simulink subsystem "HMT_Controller"  (R2022b)
settings: Solver=VariableStepAuto  StartTime=0.0  StopTime=10.0  RelTol=1e-3
libraries: simulink x1
settings Model: Creator=david  LastModifiedBy=david

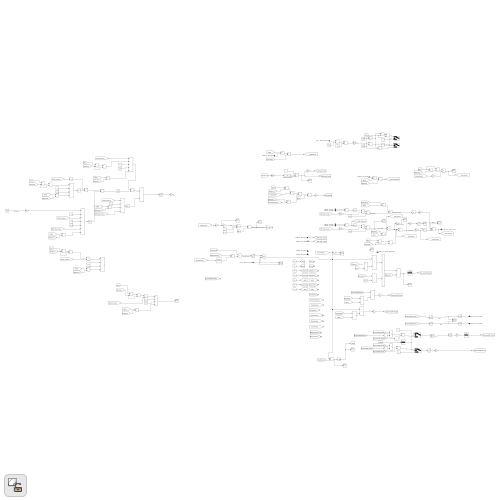
[thumbnail: Simulink's stored preview of the top-level diagram]
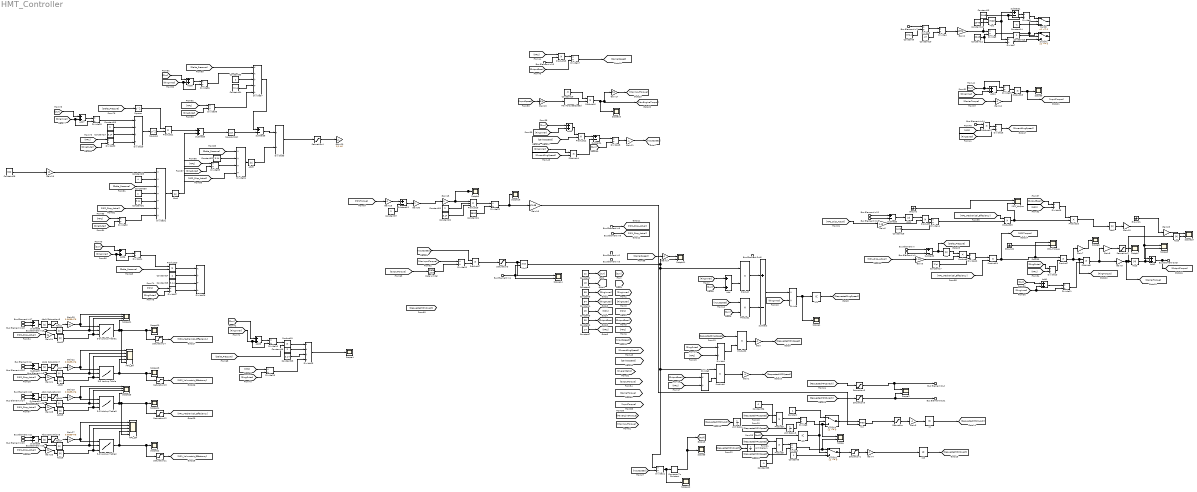
== system HMT_Controller ==
  Bus Element In{,6,12,17,21..22} (6 alike) : Inport  PortName=Feedback  Element=Pressure_A
  Bus Element In{1,10,13,18,23..24} (6 alike) : Inport  PortName=Feedback  Element=Pressure_B
  Bus Element In{2,14,25..26} (4 alike) : Inport  PortName=Feedback  Element=MP1_Speed
  Bus Element In{3,5,15,19} (4 alike) : Inport  PortName=Feedback  Element=MP2_Speed
  Bus Element In8 : Inport  PortName=Feedback  Element=MP1_Swash
  Bus Element In9 : Inport  PortName=Feedback  Element=MP2_Swash
  Bus Element In4 : Inport  Port=2  PortName=Control  Element=Speed_Command
  Bus Element In7 : Inport  Port=2  PortName=Control  Element=Speed_Command
  3-D Lookup Table : Lookup_n-D  NumberOfTableDimensions=3  BreakpointsForDimension1=[10,135,278]  BreakpointsForDimension2=[500,1974,4000]  BreakpointsForDimension3=[4.8,12,24]  Table=cat(3,[.47,0.01,0.01; .98,.38,.01;.98,.67,.38],[.81,.12,0.01;.99,.80,.65;1.00,.88,.79],[.93,.61,.42;1.00,.91,.85;1.00,.95,.89])  InterpMethod=Cubic spline  ExtrapMethod=Clip  UseLastTableValue=on  InternalRulePriority=Speed  RndMeth=Simplest
      settings: InputPortMap=u0,u1,u2
  3-D Lookup Table1 : Lookup_n-D  NumberOfTableDimensions=3  BreakpointsForDimension1=[10,135,278]  BreakpointsForDimension2=[500,1974,4000]  BreakpointsForDimension3=[4.8,12,24]  Table=cat(3,[.46,.62,.54;.27,.74,.83;.21,.73,.89],[.65,.86,.83;.46,.86,.94;.35,.86,.95],[.66,.83,.85;.53,.88,.91;.39,.87,.94])  InterpMethod=Cubic spline  ExtrapMethod=Clip  UseLastTableValue=on  InternalRulePriority=Speed  RndMeth=Simplest
      settings: InputPortMap=u0,u1,u2
  3-D Lookup Table2 : Lookup_n-D  NumberOfTableDimensions=3  BreakpointsForDimension1=[10,135,278]  BreakpointsForDimension2=[500,1974,4000]  BreakpointsForDimension3=[4.8,12,24]  Table=cat(3,[.47,0.01,0.01; .98,.38,.01;.98,.67,.38],[.81,.12,0.01;.99,.80,.65;1.00,.88,.79],[.93,.61,.42;1.00,.91,.85;1.00,.95,.89])  InterpMethod=Cubic spline  ExtrapMethod=Clip  UseLastTableValue=on  InternalRulePriority=Speed  RndMeth=Simplest
      settings: InputPortMap=u0,u1,u2
  3-D Lookup Table3 : Lookup_n-D  NumberOfTableDimensions=3  BreakpointsForDimension1=[10,135,278]  BreakpointsForDimension2=[500,1974,4000]  BreakpointsForDimension3=[4.8,12,24]  Table=cat(3,[.46,.62,.54;.27,.74,.83;.21,.73,.89],[.65,.86,.83;.46,.86,.94;.35,.86,.95],[.66,.83,.85;.53,.88,.91;.39,.87,.94])  InterpMethod=Cubic spline  ExtrapMethod=Clip  UseLastTableValue=on  InternalRulePriority=Speed  RndMeth=Simplest
      settings: InputPortMap=u0,u1,u2
  Abs{,1..18} (19 alike) : Abs  SaturateOnIntegerOverflow=off
  Add{,1..8} (9 alike) : Sum
  Compare To Constant : simulink/Logic and Bit Operations/Compare To Constant  relop=>=  const=.14389  OutDataTypeStr=boolean
  Constant : Constant
  Constant1 : Constant  Value=22
  Constant10 : Constant  Value=.27
  Constant11 : Constant  Value=2048
  Constant12 : Constant  Value=2048
  Constant13 : Constant  Value=2048
  Constant14 : Constant  Value=-1
  Constant15 : Constant
  Constant{16,20,24,26,30,33,37} (7 alike) : Constant  Value=2
  Constant17 : Constant  Value=2*pi
  Constant18 : Constant  Value=6.28
  Constant19 : Constant  Value=.8
  Constant2 : Constant  Value=18
  Constant21 : Constant  Value=3800
  Constant{22..23,25,27,31..32,34} (7 alike) : Constant  Value=3.14
  Constant28 : Constant  Value=300
  Constant29 : Constant  Value=4
  Constant3 : Constant  Value=58
  Constant35 : Constant  Value=-1
  Constant36 : Constant  Value=-1
  Constant4 : Constant  Value=54
  Constant5 : Constant  Value=25
  Constant6 : Constant  Value=38
  Constant7 : Constant  Value=14
  Constant8 : Constant
  Constant9 : Constant  Value=3724
  Divide{,1..22,24..25,27..28,30,32..33,35..36,38} (33 alike) : Product  Inputs=*/
  Divide{23,26,29,34} (4 alike) : Product  Inputs=*///
  Divide31 : Product  Inputs=***////
  Divide37 : Product  Inputs=**///
  Gain{,1,3..4,11..12,14,18} (8 alike) : Gain  Gain=-1
  Gain{8..10,23} (4 alike) : Gain  Gain=1/12
  Gain13 : Gain  Gain=3/4
  Gain15 : Gain
  Gain16 : Gain  Gain=1/1.46
  Gain17 : Gain  Gain=3/4
  Gain19 : Gain  Gain=12
  Gain2 : Gain  Gain=4096
  Gain20 : Gain  Gain=1/1.46
  Gain{21,24,26,28} (4 alike) : Gain  Gain=24
  Gain{22,25,27,29} (4 alike) : Gain  Gain=0.0689476
  Gain30 : Gain
  Gain5 : Gain  Gain=1.46
  Gain6 : Gain  Gain=1.46
  Gain7 : Gain  Gain=-1/12
  Ground : Ground
  Ground1 : Ground
  Ground2 : Ground
  IC : InitialCondition  Value=0
  IC1 : InitialCondition  Value=-1000
  IC2 : InitialCondition  Value=false
  IC3 : InitialCondition  Value=-1
  MP1_Eff : Scope  NumInputPorts=5
  MP1_Torque : Scope  NumInputPorts=2
  MP2_Eff : Scope  NumInputPorts=5
  MP2_torque : Scope  NumInputPorts=2
  MaxTorqueatSpeed : Fcn  Expr=-0.000019*u(1)^2 + 0.102035*u(1) - 80.132873
  Min : MinMax  Function=max  Inputs=2
  Min1 : MinMax  Inputs=2
  Mod : Math  Operator=mod
  Product{,1..17,19..21,23..24} (23 alike) : Product
  Product18 : Product  Inputs=3
  Rate Limiter : RateLimiter  RisingSlewLimit=inf  FallingSlewLimit=-inf  SampleTimeMode=inherited
  Saturation{,1,5..6} (4 alike) : Saturate  UpperLimit=1  LowerLimit=-1
  Saturation{7..10} (4 alike) : Saturate  UpperLimit=4000  LowerLimit=0
  Saturation{11..14} (4 alike) : Saturate  UpperLimit=1  LowerLimit=1
  Saturation2 : Saturate  UpperLimit=1000  LowerLimit=-1000
  Saturation3 : Saturate  UpperLimit=2000  LowerLimit=0
  Saturation4 : Saturate  UpperLimit=1.46  LowerLimit=-1.46
  Scope{,2,8,11,14,19} (6 alike) : Scope  NumInputPorts=2
  Scope{1,3..7,9..10,12..13,16,20,22,24} (14 alike) : Scope
  Scope21 : Scope  NumInputPorts=4
  Scope25 : Scope  NumInputPorts=4
  Square : Math  Operator=square
  Square Root : Sqrt
  Square1 : Math  Operator=square
  Subtract{,1..4,6..11} (11 alike) : Sum  Inputs=+-
  Subtract5 : Sum
  Switch : Switch  Criteria=u2 ~= 0  SaturateOnIntegerOverflow=off  InputSameDT=off
  Switch1 : Switch  Criteria=u2 ~= 0  SaturateOnIntegerOverflow=off  InputSameDT=off
  Switch2 : Switch  Criteria=u2 ~= 0  Threshold=688  SaturateOnIntegerOverflow=off  InputSameDT=off
  Switch3 : Switch  Criteria=u2 ~= 0  Threshold=688  SaturateOnIntegerOverflow=off  InputSameDT=off
  Unit Delay : UnitDelay  InitialCondition=1  SampleTime=-1  HasFrameUpgradeWarning=on
  Unit Delay1 : UnitDelay  SampleTime=-1  HasFrameUpgradeWarning=on
  Unit Delay3 : UnitDelay  InitialCondition=1  SampleTime=-1  HasFrameUpgradeWarning=on
  Bus Element Out : Outport  VectorParamsAs1DForOutWhenUnconnected=off  PortName=Control_Out  Element=MP1_Swash
  Bus Element Out1 : Outport  VectorParamsAs1DForOutWhenUnconnected=off  PortName=Control_Out  Element=MP2_Swash
  Bus Element Out2 : Outport  VectorParamsAs1DForOutWhenUnconnected=off  PortName=Control_Out  Element=Engine_Speed_CMD
  Bus Element Out3 : Outport  VectorParamsAs1DForOutWhenUnconnected=off  PortName=Control_Out  Element=Output_Torque
  wires:
  [OutputTorque] -> Rate Limiter/1
  Min1/1 -> Product/1, Product4/1, Divide21/1, Scope11/2
  Min/1 -> Saturation/1
  Saturation4/1 -> Gain20/1
  Abs5/1 -> Divide33/2
  Divide34/1 -> Abs5/1
  Abs4/1 -> Subtract5/2
  Divide37/1 -> Subtract6/1
  Subtract6/1 -> Divide33/1
  Square Root/1 -> Subtract6/2
  [MP1] -> Divide38/1
  [RingOuter] -> Divide38/2
  Divide38/1 -> Divide37/5
  Constant34/1 -> Divide37/4
  Constant33/1 -> Divide37/3
  [Delta_Pressure] -> Divide37/1
  Divide36/1 -> Divide37/2
  Add8/1 -> Divide36/1
  [RingInner] -> Divide36/2, Add8/2
  [Sun] -> Add8/1
  Gain19/1 -> Divide31/1
  Divide33/1 -> Saturation4/1
  [MP2_Disp_Actual] -> Divide34/4
  [MP1] -> Divide35/1
  [RingOuter] -> Divide35/2
  Divide35/1 -> Divide34/3
  Constant32/1 -> Divide34/2
  [Delta_Pressure] -> Divide34/1
  Subtract5/1 -> Square Root/1
  Divide31/1 -> Abs4/1
  Divide32/1 -> Divide31/7
  [RingOuter] -> Divide32/2
  [MP1] -> Divide32/1
  [MP2_Disp_Actual] -> Divide31/6
  Constant31/1 -> Divide31/5
  Constant30/1 -> Divide31/4
  Constant29/1 -> Divide31/2
  Constant28/1 -> Gain19/1  "Torque Limit"
  [Delta_Pressure] -> Divide31/3
  Product21/1 -> Subtract5/1
  Square/1 -> Product21/1
  Square1/1 -> Product21/2
  Divide29/1 -> Square1/1
  Divide28/1 -> Divide29/1
  [Sun] -> Add7/1
  [RingInner] -> Add7/2, Divide28/2
  Add7/1 -> Divide28/1
  Constant26/1 -> Divide29/2
  Constant27/1 -> Divide29/3
  Divide30/1 -> Divide29/4
  [RingOuter] -> Divide30/2
  [MP1] -> Divide30/1
  [Delta_Pressure] -> Square/1
  [MP1] -> Divide27/1
  [RingOuter] -> Divide27/2
  Divide27/1 -> Divide26/4
  Constant25/1 -> Divide26/3
  Constant24/1 -> Divide26/2
  Product20/1 -> Divide26/1
  [Delta_Pressure] -> Product20/2
  Divide24/1 -> Product20/1
  Add6/1 -> Divide24/1
  [RingInner] -> Divide24/2, Add6/2
  [Sun] -> Add6/1
  Constant1/1 -> [Sun]
  Constant2/1 -> [Planet]
  Constant4/1 -> [RingOuter]
  Constant3/1 -> [RingInner]
  Constant5/1 -> [MP1]
  Constant6/1 -> [OutputGear]
  Constant7/1 -> [MP2]
  [RingInner] -> Add/1
  [Sun] -> Add/2
  Add/1 -> Product/2
  [Sun] -> Product1/2
  Product1/1 -> Subtract/2
  Product/1 -> Subtract/1
  Subtract/1 -> Divide/1
  [RingInner] -> Divide/2
  [InputSpeed] -> Product1/1
  Divide/1 -> IC1/1, Scope1/1
  [RequestedRingSpeed] -> Product2/1
  [RingOuter] -> Divide1/1
  [MP1] -> Divide1/2
  Divide1/1 -> Product2/2
  Product2/1 -> Gain/1
  Gain/1 -> [RequestedMP1Speed]
  Divide2/1 -> Product4/2
  [OutputGear] -> Divide2/1
  [MP2] -> Divide2/2
  Gain1/1 -> [RequestedMP2Speed]
  Bus Element In7/1 -> Divide3/1
  Constant9/1 -> Divide3/2
  Constant10/1 -> Divide4/2
  Divide3/1 -> Divide4/1
  Divide4/1 -> Gain2/1
  Gain2/1 -> Mod/1, Divide5/1
  Constant11/1 -> Divide7/2, Divide5/2
  Constant12/1 -> Mod/2
  Constant13/1 -> Divide6/2, Subtract1/2
  Subtract1/1 -> Divide6/1
  Divide6/1 -> Switch/1
  Constant14/1 -> Switch/3
  Divide5/1 -> Switch/2, Switch1/2
  Constant15/1 -> Switch1/1
  Mod/1 -> Subtract1/1, Divide7/1
  Divide7/1 -> Switch1/3
  [RequestedMP2Speed] -> Product3/1
  [RequestedMP1Speed] -> Unit Delay3/1
  [RequestedMP2Speed] -> Divide9/2
  Product5/1 -> Divide9/1
  [RequestedMP1Swash] -> Unit Delay1/1
  [RequestedMP1Speed] -> Product5/1
  Constant/1 -> Switch3/1
  Divide8/1 -> Switch3/3, Scope/1
  Bus Element In9/1 -> [MP2_Disp_Actual]
  Bus Element In8/1 -> [MP1_Disp_Actual]
  Divide9/1 -> Switch2/1, Scope/2
  Constant8/1 -> Switch2/3
  [RequestedMP2Swash] -> Unit Delay/1
  Product3/1 -> Divide8/1
  Unit Delay3/1 -> Divide8/2
  Saturation/1 -> Gain3/1
  Gain3/1 -> IC/1
  Saturation1/1 -> Gain4/1
  IC1/1 -> [RequestedRingSpeed]
  [RequestedMP1Swash] -> Saturation6/1
  IC2/1 -> Switch2/2, Switch3/2
  [Half] -> IC2/1
  Gain4/1 -> IC3/1
  Bus Element In/1 -> Subtract2/1
  Bus Element In1/1 -> Subtract2/2
  Subtract2/1 -> Abs/1, [Delta_Pressure]
  Abs/1 -> Product6/1
  Add1/1 -> Divide11/1
  Gain5/1 -> Product6/2
  Product6/1 -> Divide12/1
  Constant17/1 -> Divide12/2
  Product8/1 -> Gain8/1, Gain9/1  "Carrier Torque"
  Divide13/1 -> Product7/2
  Product7/1 -> Product8/1, [RingTorque], Gain7/1  "Ring torque"
  Divide11/1 -> Product8/2
  Gain7/1 -> Scope6/1  "Ring Torque ftlb"
  [MP1] -> Divide13/2
  [RingOuter] -> Divide13/1
  Saturation2/1 -> Scope7/1
  Gain8/1 -> Saturation2/1
  [Sun] -> Add1/1
  [RingInner] -> Add1/2, Divide11/2
  Constant18/1 -> Divide14/2
  Product9/1 -> Divide14/1
  Gain6/1 -> Product9/2
  Abs1/1 -> Product9/1
  Subtract3/1 -> Abs1/1
  Bus Element In13/1 -> Subtract3/2
  Bus Element In12/1 -> Subtract3/1
  Divide14/1 -> Product23/2  "Control"
  [OutputGear] -> Divide15/1
  [MP2] -> Divide15/2
  Divide15/1 -> Product10/1
  Gain9/1 -> [CarrierTorque], Abs3/1, Abs9/1  "Carrier"
  Product10/1 -> Abs2/1  "MP2 Output Torque"
  Gain10/1 -> Add2/1, Scope8/1  "MP2"
  Abs2/1 -> Gain10/1
  Add2/1 -> Bus Element Out3/1, [OutputTorque]
  Bus Element In14/1 -> Product11/1
  [MP1] -> Product11/2
  Product11/1 -> Divide16/1
  [RingOuter] -> Divide16/2
  Divide16/1 -> [CurrentRingSpeed]
  [Sun] -> Add3/1
  [RingInner] -> Add3/2
  Add3/1 -> Product12/1
  [MP2] -> Product13/1
  Bus Element In15/1 -> Product13/2
  Product13/1 -> Divide17/1
  [OutputGear] -> Divide17/2
  [CarrierSpeed] -> Product12/2
  [CurrentRingSpeed] -> Product14/2
  [RingInner] -> Product14/1
  Product12/1 -> Subtract4/1
  Product14/1 -> Subtract4/2
  Subtract4/1 -> Divide18/1
  [Sun] -> Divide18/2
  Divide18/1 -> Gain11/1
  Gain11/1 -> [InputSpeed]
  Divide17/1 -> [CarrierSpeed]
  Add4/1 -> Divide19/2
  [RingInner] -> Add4/2
  [Sun] -> Add4/1, Divide19/1
  Abs3/1 -> Add2/2, Scope8/2
  Divide19/1 -> Product15/1
  [CarrierTorque] -> Gain12/1
  Product15/1 -> Scope9/1, [InputTorque]
  Gain12/1 -> Product15/2
  [InputSpeed] -> Gain13/1
  Gain13/1 -> MaxTorqueatSpeed/1
  Product16/1 -> [MaxEngineTorque], Gain17/1, Scope10/1
  MaxTorqueatSpeed/1 -> Product16/2  "Max Torque"
  Constant19/1 -> Product16/1
  Gain17/1 -> [MaxInputTorque]
  [MaxInputTorque] -> Divide20/1
  Divide20/1 -> Product17/2
  [InputSpeed] -> Product17/1
  Product17/1 -> Saturation3/1  "Permissible Speed"
  Bus Element In4/1 -> Min1/2, Scope14/2
  [CarrierSpeed] -> Gain14/1
  Gain14/1 -> Scope11/1
  Product4/1 -> Gain1/1
  [InputSpeed] -> Divide21/2
  Divide21/1 -> Compare To Constant/1, Scope12/1
  Compare To Constant/1 -> [Half], Scope5/1
  Saturation3/1 -> Scope14/1, Min1/1
  IC/1 -> [RequestedMP1Swash]
  [RequestedMP2Swash] -> Saturation5/1
  [MP1Torque] -> Gain18/1  "ftlb"
  Gain15/1 -> Product18/1, Scope3/1  "inlb"
  Constant20/1 -> Product18/2
  Constant22/1 -> Product18/3
  Product18/1 -> Divide22/1
  Constant21/1 -> Divide22/2
  Divide22/1 -> Scope16/1, Gain16/1  "Minimum displacement cuin/rev"
  Saturation5/1 -> Bus Element Out1/1, Scope2/2  "MP2"
  Saturation6/1 -> Bus Element Out/1, Scope2/1  "MP1"
  Divide10/1 -> Product19/1
  [Delta_Pressure] -> Product19/2
  Product19/1 -> Divide23/1
  Constant16/1 -> Divide23/2
  Constant23/1 -> Divide23/3
  Divide25/1 -> Divide23/4
  [RingOuter] -> Divide25/2
  [MP1] -> Divide25/1
  [Sun] -> Add5/1
  [RingInner] -> Add5/2, Divide10/2
  Add5/1 -> Divide10/1
  Divide23/1 -> Scope4/1
  [MP2_Disp_Actual] -> Gain21/1
  Gain21/1 -> Abs8/1
  Bus Element In5/1 -> Abs7/1
  Bus Element In6/1 -> Subtract7/1
  Bus Element In10/1 -> Subtract7/2
  Abs7/1 -> 3-D Lookup Table/2, MP2_Eff/2  "Speed"
  Abs8/1 -> 3-D Lookup Table/3, MP2_Eff/3  "Displacement"
  3-D Lookup Table/1 -> Scope13/1, Saturation13/1, MP2_Eff/4  "Volumetric Effiecency"
  Abs6/1 -> Saturation7/1  "Pressure_Drop"
  Saturation7/1 -> Gain22/1  "Pressure Drop"
  Subtract7/1 -> Abs6/1
  Gain22/1 -> MP2_Eff/1, 3-D Lookup Table/1  "Pressure_Drop"
  Ground/1 -> MP2_torque/1  "Actual"
  Ground1/1 -> Gain23/1
  Gain23/1 -> Scope19/1
  Abs9/1 -> Scope19/2
  Gain25/1 -> 3-D Lookup Table1/1, Scope21/1  "Pressure_Drop"
  Subtract8/1 -> Abs10/1
  Saturation8/1 -> Gain25/1  "Pressure Drop"
  Abs10/1 -> Saturation8/1  "Pressure_Drop"
  3-D Lookup Table1/1 -> Scope21/4, Saturation14/1, Scope20/1, MP2_Eff/5  "Mechanical Effiecency"
  Abs12/1 -> Scope21/3, 3-D Lookup Table1/3  "Displacement"
  Abs11/1 -> Scope21/2, 3-D Lookup Table1/2  "Speed"
  Bus Element In18/1 -> Subtract8/2
  Bus Element In17/1 -> Subtract8/1
  Bus Element In19/1 -> Abs11/1
  Gain24/1 -> Abs12/1
  [MP2_Disp_Actual] -> Gain24/1
  [MP2_Mechanical_Effeciency] -> Product23/1
  Product23/1 -> Product10/2, MP2_torque/2
  [MP2_Disp_Actual] -> Gain6/1
  Ground2/1 -> MP1_Torque/2  "Actual"
  [MP1_Disp_Actual] -> Gain28/1
  Gain28/1 -> Abs15/1
  Bus Element In26/1 -> Abs14/1
  Bus Element In22/1 -> Subtract10/1
  Bus Element In24/1 -> Subtract10/2
  Abs14/1 -> 3-D Lookup Table3/2, Scope25/2  "Speed"
  Abs15/1 -> 3-D Lookup Table3/3, Scope25/3  "Displacement"
  3-D Lookup Table3/1 -> Scope24/1, Saturation12/1, MP1_Eff/5, Scope25/4  "Mechanical Effiecency"
  Abs13/1 -> Saturation10/1  "Pressure_Drop"
  Saturation10/1 -> Gain29/1  "Pressure Drop"
  Subtract10/1 -> Abs13/1
  Gain29/1 -> Scope25/1, 3-D Lookup Table3/1  "Pressure_Drop"
  Gain27/1 -> 3-D Lookup Table2/1, MP1_Eff/1  "Pressure_Drop"
  Subtract9/1 -> Abs16/1
  Saturation9/1 -> Gain27/1  "Pressure Drop"
  Abs16/1 -> Saturation9/1  "Pressure_Drop"
  3-D Lookup Table2/1 -> MP1_Eff/4, Saturation11/1, Scope22/1  "Volumetric Effiecency"
  Abs18/1 -> MP1_Eff/3, 3-D Lookup Table2/3  "Displacement"
  Abs17/1 -> MP1_Eff/2, 3-D Lookup Table2/2  "Speed"
  Bus Element In23/1 -> Subtract9/2
  Bus Element In21/1 -> Subtract9/1
  Bus Element In25/1 -> Abs17/1
  Gain26/1 -> Abs18/1
  [MP1_Disp_Actual] -> Gain26/1
  Divide12/1 -> Product24/1  "MP1_Torque"
  Product24/1 -> Product7/1, MP1_Torque/1, [MP1Torque]  "Control"
  [MP1_Mechanical_Effeciency] -> Product24/2
  [MP1_Disp_Actual] -> Gain5/1
  Rate Limiter/1 -> Divide20/2
  Saturation11/1 -> [MP1_Volumetric_Effeciency]
  Saturation12/1 -> [MP1_Mechanical_Effeciency]
  Saturation13/1 -> [MP2_Volumetric_Effeciency]
  Saturation14/1 -> [MP2_Mechanical_Effeciency]
  IC3/1 -> [RequestedMP2Swash]
  Switch3/1 -> Min/1
  Switch2/1 -> Saturation1/1
  Constant35/1 -> Product5/2
  Constant36/1 -> Product3/2
  Gain18/1 -> Subtract11/1
  Subtract11/1 -> Gain30/1
  Gain30/1 -> Gain15/1
  Gain16/1 -> Min/2  "Minimum swash command"
  Constant37/1 -> Subtract11/2
